simulink library "ammclib_bam_S32K11x"  (R2016a)
settings: Solver=VariableStepAuto  SolverMode=SingleTasking  StartTime=0.0  StopTime=10.0  RelTol=1e-3
undefined symbols (not defined in the file or in its folder): f16A1, f16A2, f16ADCMaxError, f16B0, f16B1, f16B2, f16C1, f16CC1, f16CC1sc, f16CC1sc_D, f16CC1sc_Q, f16CC2, f16CC2sc, f16CC2sc_D, f16CC2sc_Q, f16DerivGain, f16EGain, f16FiltCoef, f16HystOff, f16HystOn, f16IGain, f16IntegGain, f16IntegGainFW, f16IntegGainQ, f16Kd, f16Kq, f16Limit, f16LowerLimit, f16LowerLimit_D, f16LowerLimit_Q, f16LowerLimitFW, f16LowerLimitQ, f16ModIndex, f16OutValOff, f16OutValOn, f16PropGain, f16PropGainFW, f16PropGainQ, f16RampDown, f16RampUp, f16UGain, f16UpperLimit, f16UpperLimit_D, f16UpperLimit_Q, f16UpperLimitFW, f16UpperLimitQ, f16WIGain, f32A1, f32A2, f32ADCMaxError, f32B0, f32B1, f32B2, f32C1, f32CC1, f32CC1sc, f32CC1sc_D, f32CC1sc_Q, f32CC2, f32CC2sc ... (+62)
(part 15 of 16)

== system ammclib_bam_S32K11x/MLIB/F16/MLIB_VSub_F16 ==
  f16In1 : Inport  OutDataTypeStr=Bus: SWLIBS_2Syst_F16  BusOutputAsStruct=on
  f16In2 : Inport  Port=2  OutDataTypeStr=Bus: SWLIBS_2Syst_F16  BusOutputAsStruct=on
  MLIB_VSub_SF : S-Function  FunctionName=MLIB_VSub_SF_F16  SFunctionDeploymentMode=off  EnableBusSupport=off
  copyright : Subsystem
      mask Display: text(10,90,'FILE:');text(10,75,'DESRIPTION:');text(10,60,'COPYRIGHT:');text(10,45,'VERSION:');text(10,30,'DATE:')
  copyright2 : Subsystem
      mask Display: text(10,90,'MLIB_VSub_BAM_F16.mdl');text(10,75,'Vector substraction.');text(10,60,'NXP 2020');text(10,45,'1.0');text(10,30,'01-Jun-2020');
  f16Out : Outport
  wires:
  MLIB_VSub_SF/1 -> f16Out/1
  f16In2/1 -> MLIB_VSub_SF/2
  f16In1/1 -> MLIB_VSub_SF/1

== system ammclib_bam_S32K11x/MLIB/F32/MLIB_AbsSat_F32 ==
  f32In : Inport  OutDataTypeStr=int32
  MLIB_AbsSat_SF : S-Function  FunctionName=MLIB_AbsSat_SF_F32  SFunctionDeploymentMode=off  EnableBusSupport=off
  copyright : Subsystem
      mask Display: text(10,90,'FILE:');text(10,75,'DESRIPTION:');text(10,60,'COPYRIGHT:');text(10,45,'VERSION:');text(10,30,'DATE:')
  copyright2 : Subsystem
      mask Display: text(10,90,'MLIB_AbsSat_BAM_F32.mdl');text(10,75,'Saturated absolute value.');text(10,60,'NXP 2020');text(10,45,'1.0');text(10,30,'18-Mar-2020');
  f32Out : Outport
  wires:
  MLIB_AbsSat_SF/1 -> f32Out/1
  f32In/1 -> MLIB_AbsSat_SF/1

== system ammclib_bam_S32K11x/MLIB/F32/MLIB_Abs_F32 ==
  f32In : Inport  OutDataTypeStr=int32
  MLIB_Abs_SF : S-Function  FunctionName=MLIB_Abs_SF_F32  SFunctionDeploymentMode=off  EnableBusSupport=off
  copyright : Subsystem
      mask Display: text(10,90,'FILE:');text(10,75,'DESRIPTION:');text(10,60,'COPYRIGHT:');text(10,45,'VERSION:');text(10,30,'DATE:')
  copyright2 : Subsystem
      mask Display: text(10,90,'MLIB_Abs_BAM_F32.mdl');text(10,75,'Unsaturated absolute value.');text(10,60,'NXP 2020');text(10,45,'1.0');text(10,30,'18-Mar-2020');
  f32Out : Outport
  wires:
  MLIB_Abs_SF/1 -> f32Out/1
  f32In/1 -> MLIB_Abs_SF/1

== system ammclib_bam_S32K11x/MLIB/F32/MLIB_AddSat_F32 ==
  f32In1 : Inport  OutDataTypeStr=int32
  f32In2 : Inport  Port=2  OutDataTypeStr=int32
  MLIB_AddSat_SF : S-Function  FunctionName=MLIB_AddSat_SF_F32  SFunctionDeploymentMode=off  EnableBusSupport=off
  copyright : Subsystem
      mask Display: text(10,90,'FILE:');text(10,75,'DESRIPTION:');text(10,60,'COPYRIGHT:');text(10,45,'VERSION:');text(10,30,'DATE:')
  copyright2 : Subsystem
      mask Display: text(10,90,'MLIB_AddSat_BAM_F32.mdl');text(10,75,'Saturated addition.');text(10,60,'NXP 2020');text(10,45,'1.0');text(10,30,'18-Mar-2020');
  f32Out : Outport
  wires:
  MLIB_AddSat_SF/1 -> f32Out/1
  f32In2/1 -> MLIB_AddSat_SF/2
  f32In1/1 -> MLIB_AddSat_SF/1

== system ammclib_bam_S32K11x/MLIB/F32/MLIB_Add_F32 ==
  f32In1 : Inport  OutDataTypeStr=int32
  f32In2 : Inport  Port=2  OutDataTypeStr=int32
  MLIB_Add_SF : S-Function  FunctionName=MLIB_Add_SF_F32  SFunctionDeploymentMode=off  EnableBusSupport=off
  copyright : Subsystem
      mask Display: text(10,90,'FILE:');text(10,75,'DESRIPTION:');text(10,60,'COPYRIGHT:');text(10,45,'VERSION:');text(10,30,'DATE:')
  copyright2 : Subsystem
      mask Display: text(10,90,'MLIB_Add_BAM_F32.mdl');text(10,75,'Unsaturated addition.');text(10,60,'NXP 2020');text(10,45,'1.0');text(10,30,'18-Mar-2020');
  f32Out : Outport
  wires:
  MLIB_Add_SF/1 -> f32Out/1
  f32In2/1 -> MLIB_Add_SF/2
  f32In1/1 -> MLIB_Add_SF/1

== system ammclib_bam_S32K11x/MLIB/F32/MLIB_ConvertPU_F32F16 ==
  f16In : Inport  OutDataTypeStr=int16
  MLIB_ConvertPU_SF : S-Function  FunctionName=MLIB_ConvertPU_SF_F32F16  SFunctionDeploymentMode=off  EnableBusSupport=off
  copyright : Subsystem
      mask Display: text(10,90,'FILE:');text(10,75,'DESRIPTION:');text(10,60,'COPYRIGHT:');text(10,45,'VERSION:');text(10,30,'DATE:')
  copyright2 : Subsystem
      mask Display: text(10,90,'MLIB_ConvertPU_BAM_F32F16.mdl');text(10,75,'Converts the input value to a different representation.');text(10,60,'NXP 2020');text(10,45,'1.0');text(10,30,'18-Mar-2020');
  f32Out : Outport
  wires:
  MLIB_ConvertPU_SF/1 -> f32Out/1
  f16In/1 -> MLIB_ConvertPU_SF/1

== system ammclib_bam_S32K11x/MLIB/F32/MLIB_Convert_F32F16 ==
  f16In1 : Inport  OutDataTypeStr=int16
  f16In2 : Inport  Port=2  OutDataTypeStr=int16
  MLIB_Convert_SF : S-Function  FunctionName=MLIB_Convert_SF_F32F16  SFunctionDeploymentMode=off  EnableBusSupport=off
  copyright : Subsystem
      mask Display: text(10,90,'FILE:');text(10,75,'DESRIPTION:');text(10,60,'COPYRIGHT:');text(10,45,'VERSION:');text(10,30,'DATE:')
  copyright2 : Subsystem
      mask Display: text(10,90,'MLIB_Convert_BAM_F32F16.mdl');text(10,75,'Converts the input value with scale to a different representation.');text(10,60,'NXP 2020');text(10,45,'1.0');text(10,30,'18-Mar-2020');
  f32Out : Outport
  wires:
  MLIB_Convert_SF/1 -> f32Out/1
  f16In2/1 -> MLIB_Convert_SF/2
  f16In1/1 -> MLIB_Convert_SF/1

== system ammclib_bam_S32K11x/MLIB/F32/MLIB_DivSat_F32 ==
  f32In1 : Inport  OutDataTypeStr=int32
  f32In2 : Inport  Port=2  OutDataTypeStr=int32
  MLIB_DivSat_SF : S-Function  FunctionName=MLIB_DivSat_SF_F32  SFunctionDeploymentMode=off  EnableBusSupport=off
  copyright : Subsystem
      mask Display: text(10,90,'FILE:');text(10,75,'DESRIPTION:');text(10,60,'COPYRIGHT:');text(10,45,'VERSION:');text(10,30,'DATE:')
  copyright2 : Subsystem
      mask Display: text(10,90,'MLIB_DivSat_BAM_F32.mdl');text(10,75,'Saturated division.');text(10,60,'NXP 2020');text(10,45,'1.0');text(10,30,'18-Mar-2020');
  f32Out : Outport
  wires:
  MLIB_DivSat_SF/1 -> f32Out/1
  f32In2/1 -> MLIB_DivSat_SF/2
  f32In1/1 -> MLIB_DivSat_SF/1

== system ammclib_bam_S32K11x/MLIB/F32/MLIB_Div_F32 ==
  f32In1 : Inport  OutDataTypeStr=int32
  f32In2 : Inport  Port=2  OutDataTypeStr=int32
  MLIB_Div_SF : S-Function  FunctionName=MLIB_Div_SF_F32  SFunctionDeploymentMode=off  EnableBusSupport=off
  copyright : Subsystem
      mask Display: text(10,90,'FILE:');text(10,75,'DESRIPTION:');text(10,60,'COPYRIGHT:');text(10,45,'VERSION:');text(10,30,'DATE:')
  copyright2 : Subsystem
      mask Display: text(10,90,'MLIB_Div_BAM_F32.mdl');text(10,75,'Division of two input values.');text(10,60,'NXP 2020');text(10,45,'1.0');text(10,30,'18-Mar-2020');
  f32Out : Outport
  wires:
  MLIB_Div_SF/1 -> f32Out/1
  f32In2/1 -> MLIB_Div_SF/2
  f32In1/1 -> MLIB_Div_SF/1

== system ammclib_bam_S32K11x/MLIB/F32/MLIB_MacSat_F32 ==
  f32In1 : Inport  OutDataTypeStr=int32
  f32In2 : Inport  Port=2  OutDataTypeStr=int32
  f32In3 : Inport  Port=3  OutDataTypeStr=int32
  MLIB_MacSat_SF : S-Function  FunctionName=MLIB_MacSat_SF_F32  SFunctionDeploymentMode=off  EnableBusSupport=off
  copyright : Subsystem
      mask Display: text(10,90,'FILE:');text(10,75,'DESRIPTION:');text(10,60,'COPYRIGHT:');text(10,45,'VERSION:');text(10,30,'DATE:')
  copyright2 : Subsystem
      mask Display: text(10,90,'MLIB_MacSat_BAM_F32.mdl');text(10,75,'Saturated multiply-accumulate.');text(10,60,'NXP 2020');text(10,45,'1.0');text(10,30,'18-Mar-2020');
  f32Out : Outport
  wires:
  MLIB_MacSat_SF/1 -> f32Out/1
  f32In3/1 -> MLIB_MacSat_SF/3
  f32In2/1 -> MLIB_MacSat_SF/2
  f32In1/1 -> MLIB_MacSat_SF/1

== system ammclib_bam_S32K11x/MLIB/F32/MLIB_Mac_F32 ==
  f32In1 : Inport  OutDataTypeStr=int32
  f32In2 : Inport  Port=2  OutDataTypeStr=int32
  f32In3 : Inport  Port=3  OutDataTypeStr=int32
  MLIB_Mac_SF : S-Function  FunctionName=MLIB_Mac_SF_F32  SFunctionDeploymentMode=off  EnableBusSupport=off
  copyright : Subsystem
      mask Display: text(10,90,'FILE:');text(10,75,'DESRIPTION:');text(10,60,'COPYRIGHT:');text(10,45,'VERSION:');text(10,30,'DATE:')
  copyright2 : Subsystem
      mask Display: text(10,90,'MLIB_Mac_BAM_F32.mdl');text(10,75,'Multiply-accumulte.');text(10,60,'NXP 2020');text(10,45,'1.0');text(10,30,'18-Mar-2020');
  f32Out : Outport
  wires:
  MLIB_Mac_SF/1 -> f32Out/1
  f32In3/1 -> MLIB_Mac_SF/3
  f32In2/1 -> MLIB_Mac_SF/2
  f32In1/1 -> MLIB_Mac_SF/1

== system ammclib_bam_S32K11x/MLIB/F32/MLIB_Mnac_F32 ==
  f32In1 : Inport  OutDataTypeStr=int32
  f32In2 : Inport  Port=2  OutDataTypeStr=int32
  f32In3 : Inport  Port=3  OutDataTypeStr=int32
  MLIB_Mnac_SF : S-Function  FunctionName=MLIB_Mnac_SF_F32  SFunctionDeploymentMode=off  EnableBusSupport=off
  copyright : Subsystem
      mask Display: text(10,90,'FILE:');text(10,75,'DESRIPTION:');text(10,60,'COPYRIGHT:');text(10,45,'VERSION:');text(10,30,'DATE:')
  copyright2 : Subsystem
      mask Display: text(10,90,'MLIB_Mnac_BAM_F32.mdl');text(10,75,'Unsaturated multiply-negative-accumulate.');text(10,60,'NXP 2020');text(10,45,'1.0');text(10,30,'18-Mar-2020');
  f32Out : Outport
  wires:
  MLIB_Mnac_SF/1 -> f32Out/1
  f32In3/1 -> MLIB_Mnac_SF/3
  f32In2/1 -> MLIB_Mnac_SF/2
  f32In1/1 -> MLIB_Mnac_SF/1

== system ammclib_bam_S32K11x/MLIB/F32/MLIB_Msu_F32 ==
  f32In1 : Inport  OutDataTypeStr=int32
  f32In2 : Inport  Port=2  OutDataTypeStr=int32
  f32In3 : Inport  Port=3  OutDataTypeStr=int32
  MLIB_Msu_SF : S-Function  FunctionName=MLIB_Msu_SF_F32  SFunctionDeploymentMode=off  EnableBusSupport=off
  copyright : Subsystem
      mask Display: text(10,90,'FILE:');text(10,75,'DESRIPTION:');text(10,60,'COPYRIGHT:');text(10,45,'VERSION:');text(10,30,'DATE:')
  copyright2 : Subsystem
      mask Display: text(10,90,'MLIB_Msu_BAM_F32.mdl');text(10,75,'Unsaturated multiply-subtract-from.');text(10,60,'NXP 2020');text(10,45,'1.0');text(10,30,'18-Mar-2020');
  f32Out : Outport
  wires:
  MLIB_Msu_SF/1 -> f32Out/1
  f32In3/1 -> MLIB_Msu_SF/3
  f32In2/1 -> MLIB_Msu_SF/2
  f32In1/1 -> MLIB_Msu_SF/1

== system ammclib_bam_S32K11x/MLIB/F32/MLIB_MulSat_F32 ==
  f32In1 : Inport  OutDataTypeStr=int32
  f32In2 : Inport  Port=2  OutDataTypeStr=int32
  MLIB_MulSat_SF : S-Function  FunctionName=MLIB_MulSat_SF_F32  SFunctionDeploymentMode=off  EnableBusSupport=off
  copyright : Subsystem
      mask Display: text(10,90,'FILE:');text(10,75,'DESRIPTION:');text(10,60,'COPYRIGHT:');text(10,45,'VERSION:');text(10,30,'DATE:')
  copyright2 : Subsystem
      mask Display: text(10,90,'MLIB_MulSat_BAM_F32.mdl');text(10,75,'Saturated multiplication.');text(10,60,'NXP 2020');text(10,45,'1.0');text(10,30,'18-Mar-2020');
  f32Out : Outport
  wires:
  MLIB_MulSat_SF/1 -> f32Out/1
  f32In2/1 -> MLIB_MulSat_SF/2
  f32In1/1 -> MLIB_MulSat_SF/1

== system ammclib_bam_S32K11x/MLIB/F32/MLIB_Mul_F32 ==
  f32In1 : Inport  OutDataTypeStr=int32
  f32In2 : Inport  Port=2  OutDataTypeStr=int32
  MLIB_Mul_SF : S-Function  FunctionName=MLIB_Mul_SF_F32  SFunctionDeploymentMode=off  EnableBusSupport=off
  copyright : Subsystem
      mask Display: text(10,90,'FILE:');text(10,75,'DESRIPTION:');text(10,60,'COPYRIGHT:');text(10,45,'VERSION:');text(10,30,'DATE:')
  copyright2 : Subsystem
      mask Display: text(10,90,'MLIB_Mul_BAM_F32.mdl');text(10,75,'Unsaturated multiplication.');text(10,60,'NXP 2020');text(10,45,'1.0');text(10,30,'18-Mar-2020');
  f32Out : Outport
  wires:
  MLIB_Mul_SF/1 -> f32Out/1
  f32In2/1 -> MLIB_Mul_SF/2
  f32In1/1 -> MLIB_Mul_SF/1

== system ammclib_bam_S32K11x/MLIB/F32/MLIB_NegSat_F32 ==
  f32In : Inport  OutDataTypeStr=int32
  MLIB_NegSat_SF : S-Function  FunctionName=MLIB_NegSat_SF_F32  SFunctionDeploymentMode=off  EnableBusSupport=off
  copyright : Subsystem
      mask Display: text(10,90,'FILE:');text(10,75,'DESRIPTION:');text(10,60,'COPYRIGHT:');text(10,45,'VERSION:');text(10,30,'DATE:')
  copyright2 : Subsystem
      mask Display: text(10,90,'MLIB_NegSat_BAM_F32.mdl');text(10,75,'Saturated negation.');text(10,60,'NXP 2020');text(10,45,'1.0');text(10,30,'18-Mar-2020');
  f32Out : Outport
  wires:
  MLIB_NegSat_SF/1 -> f32Out/1
  f32In/1 -> MLIB_NegSat_SF/1

== system ammclib_bam_S32K11x/MLIB/F32/MLIB_Neg_F32 ==
  f32In : Inport  OutDataTypeStr=int32
  MLIB_Neg_SF : S-Function  FunctionName=MLIB_Neg_SF_F32  SFunctionDeploymentMode=off  EnableBusSupport=off
  copyright : Subsystem
      mask Display: text(10,90,'FILE:');text(10,75,'DESRIPTION:');text(10,60,'COPYRIGHT:');text(10,45,'VERSION:');text(10,30,'DATE:')
  copyright2 : Subsystem
      mask Display: text(10,90,'MLIB_Neg_BAM_F32.mdl');text(10,75,'Unsaturated negation.');text(10,60,'NXP 2020');text(10,45,'1.0');text(10,30,'18-Mar-2020');
  f32Out : Outport
  wires:
  MLIB_Neg_SF/1 -> f32Out/1
  f32In/1 -> MLIB_Neg_SF/1

== system ammclib_bam_S32K11x/MLIB/F32/MLIB_Norm_F32 ==
  f32In : Inport  OutDataTypeStr=int32
  MLIB_Norm_SF : S-Function  FunctionName=MLIB_Norm_SF_F32  SFunctionDeploymentMode=off  EnableBusSupport=off
  copyright : Subsystem
      mask Display: text(10,90,'FILE:');text(10,75,'DESRIPTION:');text(10,60,'COPYRIGHT:');text(10,45,'VERSION:');text(10,30,'DATE:')
  copyright2 : Subsystem
      mask Display: text(10,90,'MLIB_Norm_BAM_F32.mdl');text(10,75,'Normalization of the input value.');text(10,60,'NXP 2020');text(10,45,'1.0');text(10,30,'18-Mar-2020');
  u16Out : Outport
  wires:
  MLIB_Norm_SF/1 -> u16Out/1
  f32In/1 -> MLIB_Norm_SF/1

== system ammclib_bam_S32K11x/MLIB/F32/MLIB_Round_F32 ==
  f32In1 : Inport  OutDataTypeStr=int32
  u16In2 : Inport  Port=2  OutDataTypeStr=uint16
  MLIB_Round_SF : S-Function  FunctionName=MLIB_Round_SF_F32  SFunctionDeploymentMode=off  EnableBusSupport=off
  copyright : Subsystem
      mask Display: text(10,90,'FILE:');text(10,75,'DESRIPTION:');text(10,60,'COPYRIGHT:');text(10,45,'VERSION:');text(10,30,'DATE:')
  copyright2 : Subsystem
      mask Display: text(10,90,'MLIB_Round_BAM_F32.mdl');text(10,75,'Round the first input value.');text(10,60,'NXP 2020');text(10,45,'1.0');text(10,30,'18-Mar-2020');
  f32Out : Outport
  wires:
  MLIB_Round_SF/1 -> f32Out/1
  u16In2/1 -> MLIB_Round_SF/2
  f32In1/1 -> MLIB_Round_SF/1

== system ammclib_bam_S32K11x/MLIB/F32/MLIB_ShBiSat_F32 ==
  f32In1 : Inport  OutDataTypeStr=int32
  s16In2 : Inport  Port=2  OutDataTypeStr=int16
  MLIB_ShBiSat_SF : S-Function  FunctionName=MLIB_ShBiSat_SF_F32  SFunctionDeploymentMode=off  EnableBusSupport=off
  copyright : Subsystem
      mask Display: text(10,90,'FILE:');text(10,75,'DESRIPTION:');text(10,60,'COPYRIGHT:');text(10,45,'VERSION:');text(10,30,'DATE:')
  copyright2 : Subsystem
      mask Display: text(10,90,'MLIB_ShBiSat_BAM_F32.mdl');text(10,75,'Saturated bidirectional shift.');text(10,60,'NXP 2020');text(10,45,'1.0');text(10,30,'18-Mar-2020');
  f32Out : Outport
  wires:
  MLIB_ShBiSat_SF/1 -> f32Out/1
  s16In2/1 -> MLIB_ShBiSat_SF/2
  f32In1/1 -> MLIB_ShBiSat_SF/1

== system ammclib_bam_S32K11x/MLIB/F32/MLIB_ShBi_F32 ==
  f32In1 : Inport  OutDataTypeStr=int32
  s16In2 : Inport  Port=2  OutDataTypeStr=int16
  MLIB_ShBi_SF : S-Function  FunctionName=MLIB_ShBi_SF_F32  SFunctionDeploymentMode=off  EnableBusSupport=off
  copyright : Subsystem
      mask Display: text(10,90,'FILE:');text(10,75,'DESRIPTION:');text(10,60,'COPYRIGHT:');text(10,45,'VERSION:');text(10,30,'DATE:')
  copyright2 : Subsystem
      mask Display: text(10,90,'MLIB_ShBi_BAM_F32.mdl');text(10,75,'Unsaturated bidirectional shift.');text(10,60,'NXP 2020');text(10,45,'1.0');text(10,30,'18-Mar-2020');
  f32Out : Outport
  wires:
  MLIB_ShBi_SF/1 -> f32Out/1
  s16In2/1 -> MLIB_ShBi_SF/2
  f32In1/1 -> MLIB_ShBi_SF/1

== system ammclib_bam_S32K11x/MLIB/F32/MLIB_ShLSat_F32 ==
  f32In1 : Inport  OutDataTypeStr=int32
  u16In2 : Inport  Port=2  OutDataTypeStr=uint16
  MLIB_ShLSat_SF : S-Function  FunctionName=MLIB_ShLSat_SF_F32  SFunctionDeploymentMode=off  EnableBusSupport=off
  copyright : Subsystem
      mask Display: text(10,90,'FILE:');text(10,75,'DESRIPTION:');text(10,60,'COPYRIGHT:');text(10,45,'VERSION:');text(10,30,'DATE:')
  copyright2 : Subsystem
      mask Display: text(10,90,'MLIB_ShLSat_BAM_F32.mdl');text(10,75,'Saturated shift left.');text(10,60,'NXP 2020');text(10,45,'1.0');text(10,30,'18-Mar-2020');
  f32Out : Outport
  wires:
  MLIB_ShLSat_SF/1 -> f32Out/1
  u16In2/1 -> MLIB_ShLSat_SF/2
  f32In1/1 -> MLIB_ShLSat_SF/1

== system ammclib_bam_S32K11x/MLIB/F32/MLIB_ShL_F32 ==
  f32In1 : Inport  OutDataTypeStr=int32
  u16In2 : Inport  Port=2  OutDataTypeStr=uint16
  MLIB_ShL_SF : S-Function  FunctionName=MLIB_ShL_SF_F32  SFunctionDeploymentMode=off  EnableBusSupport=off
  copyright : Subsystem
      mask Display: text(10,90,'FILE:');text(10,75,'DESRIPTION:');text(10,60,'COPYRIGHT:');text(10,45,'VERSION:');text(10,30,'DATE:')
  copyright2 : Subsystem
      mask Display: text(10,90,'MLIB_ShL_BAM_F32.mdl');text(10,75,'Unsaturated shift left.');text(10,60,'NXP 2020');text(10,45,'1.0');text(10,30,'18-Mar-2020');
  f32Out : Outport
  wires:
  MLIB_ShL_SF/1 -> f32Out/1
  u16In2/1 -> MLIB_ShL_SF/2
  f32In1/1 -> MLIB_ShL_SF/1

== system ammclib_bam_S32K11x/MLIB/F32/MLIB_ShR_F32 ==
  f32In1 : Inport  OutDataTypeStr=int32
  u16In2 : Inport  Port=2  OutDataTypeStr=uint16
  MLIB_ShR_SF : S-Function  FunctionName=MLIB_ShR_SF_F32  SFunctionDeploymentMode=off  EnableBusSupport=off
  copyright : Subsystem
      mask Display: text(10,90,'FILE:');text(10,75,'DESRIPTION:');text(10,60,'COPYRIGHT:');text(10,45,'VERSION:');text(10,30,'DATE:')
  copyright2 : Subsystem
      mask Display: text(10,90,'MLIB_ShR_BAM_F32.mdl');text(10,75,'Unsaturated shift right.');text(10,60,'NXP 2020');text(10,45,'1.0');text(10,30,'18-Mar-2020');
  f32Out : Outport
  wires:
  MLIB_ShR_SF/1 -> f32Out/1
  u16In2/1 -> MLIB_ShR_SF/2
  f32In1/1 -> MLIB_ShR_SF/1

== system ammclib_bam_S32K11x/MLIB/F32/MLIB_SubSat_F32 ==
  f32In1 : Inport  OutDataTypeStr=int32
  f32In2 : Inport  Port=2  OutDataTypeStr=int32
  MLIB_SubSat_SF : S-Function  FunctionName=MLIB_SubSat_SF_F32  SFunctionDeploymentMode=off  EnableBusSupport=off
  copyright : Subsystem
      mask Display: text(10,90,'FILE:');text(10,75,'DESRIPTION:');text(10,60,'COPYRIGHT:');text(10,45,'VERSION:');text(10,30,'DATE:')
  copyright2 : Subsystem
      mask Display: text(10,90,'MLIB_SubSat_BAM_F32.mdl');text(10,75,'Saturated subtraction.');text(10,60,'NXP 2020');text(10,45,'1.0');text(10,30,'18-Mar-2020');
  f32Out : Outport
  wires:
  MLIB_SubSat_SF/1 -> f32Out/1
  f32In2/1 -> MLIB_SubSat_SF/2
  f32In1/1 -> MLIB_SubSat_SF/1

== system ammclib_bam_S32K11x/MLIB/F32/MLIB_Sub_F32 ==
  f32In1 : Inport  OutDataTypeStr=int32
  f32In2 : Inport  Port=2  OutDataTypeStr=int32
  MLIB_Sub_SF : S-Function  FunctionName=MLIB_Sub_SF_F32  SFunctionDeploymentMode=off  EnableBusSupport=off
  copyright : Subsystem
      mask Display: text(10,90,'FILE:');text(10,75,'DESRIPTION:');text(10,60,'COPYRIGHT:');text(10,45,'VERSION:');text(10,30,'DATE:')
  copyright2 : Subsystem
      mask Display: text(10,90,'MLIB_Sub_BAM_F32.mdl');text(10,75,'Unsaturated subtraction.');text(10,60,'NXP 2020');text(10,45,'1.0');text(10,30,'18-Mar-2020');
  f32Out : Outport
  wires:
  MLIB_Sub_SF/1 -> f32Out/1
  f32In2/1 -> MLIB_Sub_SF/2
  f32In1/1 -> MLIB_Sub_SF/1

== system ammclib_bam_S32K11x/MLIB/F32/MLIB_VAdd_F32 ==
  f32In1 : Inport  OutDataTypeStr=Bus: SWLIBS_2Syst_F32  BusOutputAsStruct=on
  f32In2 : Inport  Port=2  OutDataTypeStr=Bus: SWLIBS_2Syst_F32  BusOutputAsStruct=on
  MLIB_VAdd_SF : S-Function  FunctionName=MLIB_VAdd_SF_F32  SFunctionDeploymentMode=off  EnableBusSupport=off
  copyright : Subsystem
      mask Display: text(10,90,'FILE:');text(10,75,'DESRIPTION:');text(10,60,'COPYRIGHT:');text(10,45,'VERSION:');text(10,30,'DATE:')
  copyright2 : Subsystem
      mask Display: text(10,90,'MLIB_VAdd_BAM_F32.mdl');text(10,75,'Vector addition.');text(10,60,'NXP 2020');text(10,45,'1.0');text(10,30,'28-May-2020');
  f32Out : Outport
  wires:
  MLIB_VAdd_SF/1 -> f32Out/1
  f32In2/1 -> MLIB_VAdd_SF/2
  f32In1/1 -> MLIB_VAdd_SF/1

== system ammclib_bam_S32K11x/MLIB/F32/MLIB_VMac_F32 ==
  f32In1 : Inport  OutDataTypeStr=int32
  f32In2 : Inport  Port=2  OutDataTypeStr=int32
  f32In3 : Inport  Port=3  OutDataTypeStr=int32
  f32In4 : Inport  Port=4  OutDataTypeStr=int32
  MLIB_VMac_SF : S-Function  FunctionName=MLIB_VMac_SF_F32  SFunctionDeploymentMode=off  EnableBusSupport=off
  copyright : Subsystem
      mask Display: text(10,90,'FILE:');text(10,75,'DESRIPTION:');text(10,60,'COPYRIGHT:');text(10,45,'VERSION:');text(10,30,'DATE:')
  copyright2 : Subsystem
      mask Display: text(10,90,'MLIB_VMac_BAM_F32.mdl');text(10,75,'Dot product of 2-element vectors with saturated multiplication and modulo accumulation.');text(10,60,'NXP 2020');text(10,45,'1.0');text(10,30,'18-Mar-2020');
  f32Out : Outport
  wires:
  MLIB_VMac_SF/1 -> f32Out/1
  f32In4/1 -> MLIB_VMac_SF/4
  f32In3/1 -> MLIB_VMac_SF/3
  f32In2/1 -> MLIB_VMac_SF/2
  f32In1/1 -> MLIB_VMac_SF/1

== system ammclib_bam_S32K11x/MLIB/F32/MLIB_VScale_F32 ==
  f32InVec : Inport  OutDataTypeStr=Bus: SWLIBS_2Syst_F32  BusOutputAsStruct=on
  f32InScale : Inport  Port=2  OutDataTypeStr=int32
  MLIB_VScale_SF : S-Function  FunctionName=MLIB_VScale_SF_F32  SFunctionDeploymentMode=off  EnableBusSupport=off
  copyright : Subsystem
      mask Display: text(10,90,'FILE:');text(10,75,'DESRIPTION:');text(10,60,'COPYRIGHT:');text(10,45,'VERSION:');text(10,30,'DATE:')
  copyright2 : Subsystem
      mask Display: text(10,90,'MLIB_VScale_BAM_F32.mdl');text(10,75,'Multiplication of a vector and scalar.');text(10,60,'NXP 2020');text(10,45,'1.0');text(10,30,'03-Jun-2020');
  f32OutVec : Outport
  wires:
  MLIB_VScale_SF/1 -> f32OutVec/1
  f32InScale/1 -> MLIB_VScale_SF/2
  f32InVec/1 -> MLIB_VScale_SF/1

== system ammclib_bam_S32K11x/MLIB/F32/MLIB_VSub_F32 ==
  f32In1 : Inport  OutDataTypeStr=Bus: SWLIBS_2Syst_F32  BusOutputAsStruct=on
  f32In2 : Inport  Port=2  OutDataTypeStr=Bus: SWLIBS_2Syst_F32  BusOutputAsStruct=on
  MLIB_VSub_SF : S-Function  FunctionName=MLIB_VSub_SF_F32  SFunctionDeploymentMode=off  EnableBusSupport=off
  copyright : Subsystem
      mask Display: text(10,90,'FILE:');text(10,75,'DESRIPTION:');text(10,60,'COPYRIGHT:');text(10,45,'VERSION:');text(10,30,'DATE:')
  copyright2 : Subsystem
      mask Display: text(10,90,'MLIB_VSub_BAM_F32.mdl');text(10,75,'Vector substraction.');text(10,60,'NXP 2020');text(10,45,'1.0');text(10,30,'01-Jun-2020');
  f32Out : Outport
  wires:
  MLIB_VSub_SF/1 -> f32Out/1
  f32In2/1 -> MLIB_VSub_SF/2
  f32In1/1 -> MLIB_VSub_SF/1

== system ammclib_bam_S32K11x/MLIB/F32F16F16/MLIB_MacSat_F32F16F16 ==
  f32In1 : Inport  OutDataTypeStr=int32
  f16In2 : Inport  Port=2  OutDataTypeStr=int16
  f16In3 : Inport  Port=3  OutDataTypeStr=int16
  MLIB_MacSat_SF : S-Function  FunctionName=MLIB_MacSat_SF_F32F16F16  SFunctionDeploymentMode=off  EnableBusSupport=off
  copyright : Subsystem
      mask Display: text(10,90,'FILE:');text(10,75,'DESRIPTION:');text(10,60,'COPYRIGHT:');text(10,45,'VERSION:');text(10,30,'DATE:')
  copyright2 : Subsystem
      mask Display: text(10,90,'MLIB_MacSat_BAM_F32F16F16.mdl');text(10,75,'Saturated multiply-accumulate.');text(10,60,'NXP 2020');text(10,45,'1.0');text(10,30,'18-Mar-2020');
  f32Out : Outport
  wires:
  MLIB_MacSat_SF/1 -> f32Out/1
  f16In3/1 -> MLIB_MacSat_SF/3
  f16In2/1 -> MLIB_MacSat_SF/2
  f32In1/1 -> MLIB_MacSat_SF/1

== system ammclib_bam_S32K11x/MLIB/F32F16F16/MLIB_Mac_F32F16F16 ==
  f32In1 : Inport  OutDataTypeStr=int32
  f16In2 : Inport  Port=2  OutDataTypeStr=int16
  f16In3 : Inport  Port=3  OutDataTypeStr=int16
  MLIB_Mac_SF : S-Function  FunctionName=MLIB_Mac_SF_F32F16F16  SFunctionDeploymentMode=off  EnableBusSupport=off
  copyright : Subsystem
      mask Display: text(10,90,'FILE:');text(10,75,'DESRIPTION:');text(10,60,'COPYRIGHT:');text(10,45,'VERSION:');text(10,30,'DATE:')
  copyright2 : Subsystem
      mask Display: text(10,90,'MLIB_Mac_BAM_F32F16F16.mdl');text(10,75,'Multiply-accumulte.');text(10,60,'NXP 2020');text(10,45,'1.0');text(10,30,'18-Mar-2020');
  f32Out : Outport
  wires:
  MLIB_Mac_SF/1 -> f32Out/1
  f16In3/1 -> MLIB_Mac_SF/3
  f16In2/1 -> MLIB_Mac_SF/2
  f32In1/1 -> MLIB_Mac_SF/1

== system ammclib_bam_S32K11x/MLIB/F32F16F16/MLIB_Mnac_F32F16F16 ==
  f32In1 : Inport  OutDataTypeStr=int32
  f16In2 : Inport  Port=2  OutDataTypeStr=int16
  f16In3 : Inport  Port=3  OutDataTypeStr=int16
  MLIB_Mnac_SF : S-Function  FunctionName=MLIB_Mnac_SF_F32F16F16  SFunctionDeploymentMode=off  EnableBusSupport=off
  copyright : Subsystem
      mask Display: text(10,90,'FILE:');text(10,75,'DESRIPTION:');text(10,60,'COPYRIGHT:');text(10,45,'VERSION:');text(10,30,'DATE:')
  copyright2 : Subsystem
      mask Display: text(10,90,'MLIB_Mnac_BAM_F32F16F16.mdl');text(10,75,'Unsaturated multiply-negative-accumulate.');text(10,60,'NXP 2020');text(10,45,'1.0');text(10,30,'18-Mar-2020');
  f32Out : Outport
  wires:
  MLIB_Mnac_SF/1 -> f32Out/1
  f16In3/1 -> MLIB_Mnac_SF/3
  f16In2/1 -> MLIB_Mnac_SF/2
  f32In1/1 -> MLIB_Mnac_SF/1

== system ammclib_bam_S32K11x/MLIB/F32F16F16/MLIB_Msu_F32F16F16 ==
  f32In1 : Inport  OutDataTypeStr=int32
  f16In2 : Inport  Port=2  OutDataTypeStr=int16
  f16In3 : Inport  Port=3  OutDataTypeStr=int16
  MLIB_Msu_SF : S-Function  FunctionName=MLIB_Msu_SF_F32F16F16  SFunctionDeploymentMode=off  EnableBusSupport=off
  copyright : Subsystem
      mask Display: text(10,90,'FILE:');text(10,75,'DESRIPTION:');text(10,60,'COPYRIGHT:');text(10,45,'VERSION:');text(10,30,'DATE:')
  copyright2 : Subsystem
      mask Display: text(10,90,'MLIB_Msu_BAM_F32F16F16.mdl');text(10,75,'Unsaturated multiply-subtract-from.');text(10,60,'NXP 2020');text(10,45,'1.0');text(10,30,'18-Mar-2020');
  f32Out : Outport
  wires:
  MLIB_Msu_SF/1 -> f32Out/1
  f16In3/1 -> MLIB_Msu_SF/3
  f16In2/1 -> MLIB_Msu_SF/2
  f32In1/1 -> MLIB_Msu_SF/1

== system ammclib_bam_S32K11x/MLIB/F32F16F16/MLIB_MulSat_F32F16F16 ==
  f16In1 : Inport  OutDataTypeStr=int16
  f16In2 : Inport  Port=2  OutDataTypeStr=int16
  MLIB_MulSat_SF : S-Function  FunctionName=MLIB_MulSat_SF_F32F16F16  SFunctionDeploymentMode=off  EnableBusSupport=off
  copyright : Subsystem
      mask Display: text(10,90,'FILE:');text(10,75,'DESRIPTION:');text(10,60,'COPYRIGHT:');text(10,45,'VERSION:');text(10,30,'DATE:')
  copyright2 : Subsystem
      mask Display: text(10,90,'MLIB_MulSat_BAM_F32F16F16.mdl');text(10,75,'Saturated multiplication.');text(10,60,'NXP 2020');text(10,45,'1.0');text(10,30,'18-Mar-2020');
  f32Out : Outport
  wires:
  MLIB_MulSat_SF/1 -> f32Out/1
  f16In2/1 -> MLIB_MulSat_SF/2
  f16In1/1 -> MLIB_MulSat_SF/1

== system ammclib_bam_S32K11x/MLIB/F32F16F16/MLIB_Mul_F32F16F16 ==
  f16In1 : Inport  OutDataTypeStr=int16
  f16In2 : Inport  Port=2  OutDataTypeStr=int16
  MLIB_Mul_SF : S-Function  FunctionName=MLIB_Mul_SF_F32F16F16  SFunctionDeploymentMode=off  EnableBusSupport=off
  copyright : Subsystem
      mask Display: text(10,90,'FILE:');text(10,75,'DESRIPTION:');text(10,60,'COPYRIGHT:');text(10,45,'VERSION:');text(10,30,'DATE:')
  copyright2 : Subsystem
      mask Display: text(10,90,'MLIB_Mul_BAM_F32F16F16.mdl');text(10,75,'Unsaturated multiplication.');text(10,60,'NXP 2020');text(10,45,'1.0');text(10,30,'18-Mar-2020');
  f32Out : Outport
  wires:
  MLIB_Mul_SF/1 -> f32Out/1
  f16In2/1 -> MLIB_Mul_SF/2
  f16In1/1 -> MLIB_Mul_SF/1

== system ammclib_bam_S32K11x/MLIB/F32F16F16/MLIB_VMac_F32F16F16 ==
  f16In1 : Inport  OutDataTypeStr=int16
  f16In2 : Inport  Port=2  OutDataTypeStr=int16
  f16In3 : Inport  Port=3  OutDataTypeStr=int16
  f16In4 : Inport  Port=4  OutDataTypeStr=int16
  MLIB_VMac_SF : S-Function  FunctionName=MLIB_VMac_SF_F32F16F16  SFunctionDeploymentMode=off  EnableBusSupport=off
  copyright : Subsystem
      mask Display: text(10,90,'FILE:');text(10,75,'DESRIPTION:');text(10,60,'COPYRIGHT:');text(10,45,'VERSION:');text(10,30,'DATE:')
  copyright2 : Subsystem
      mask Display: text(10,90,'MLIB_VMac_BAM_F32F16F16.mdl');text(10,75,'Dot product of 2-element vectors with saturated multiplication and modulo accumulation.');text(10,60,'NXP 2020');text(10,45,'1.0');text(10,30,'18-Mar-2020');
  f32Out : Outport
  wires:
  MLIB_VMac_SF/1 -> f32Out/1
  f16In4/1 -> MLIB_VMac_SF/4
  f16In3/1 -> MLIB_VMac_SF/3
  f16In2/1 -> MLIB_VMac_SF/2
  f16In1/1 -> MLIB_VMac_SF/1

== system ammclib_bam_S32K11x/AMCLIB/F16/AMCLIB_BemfObsrvDQ_F16/copyright ==

== system ammclib_bam_S32K11x/AMCLIB/F16/AMCLIB_BemfObsrvDQ_F16/copyright2 ==

== system ammclib_bam_S32K11x/AMCLIB/F16/AMCLIB_CurrentLoop_F16/copyright ==

== system ammclib_bam_S32K11x/AMCLIB/F16/AMCLIB_CurrentLoop_F16/copyright2 ==

== system ammclib_bam_S32K11x/AMCLIB/F16/AMCLIB_FWSpeedLoop_F16/copyright ==

== system ammclib_bam_S32K11x/AMCLIB/F16/AMCLIB_FWSpeedLoop_F16/copyright2 ==

== system ammclib_bam_S32K11x/AMCLIB/F16/AMCLIB_FW_F16/copyright ==

== system ammclib_bam_S32K11x/AMCLIB/F16/AMCLIB_FW_F16/copyright2 ==

== system ammclib_bam_S32K11x/AMCLIB/F16/AMCLIB_SpeedLoop_F16/copyright ==

== system ammclib_bam_S32K11x/AMCLIB/F16/AMCLIB_SpeedLoop_F16/copyright2 ==

== system ammclib_bam_S32K11x/AMCLIB/F16/AMCLIB_TrackObsrv_F16/copyright ==

== system ammclib_bam_S32K11x/AMCLIB/F16/AMCLIB_TrackObsrv_F16/copyright2 ==

== system ammclib_bam_S32K11x/AMCLIB/F16/AMCLIB_Windmilling_F16/copyright ==

== system ammclib_bam_S32K11x/AMCLIB/F16/AMCLIB_Windmilling_F16/copyright2 ==

== system ammclib_bam_S32K11x/AMCLIB/F32/AMCLIB_BemfObsrvDQ_F32/copyright ==

== system ammclib_bam_S32K11x/AMCLIB/F32/AMCLIB_BemfObsrvDQ_F32/copyright2 ==

== system ammclib_bam_S32K11x/AMCLIB/F32/AMCLIB_CurrentLoop_F32/copyright ==

== system ammclib_bam_S32K11x/AMCLIB/F32/AMCLIB_CurrentLoop_F32/copyright2 ==

== system ammclib_bam_S32K11x/AMCLIB/F32/AMCLIB_FWSpeedLoop_F32/copyright ==

== system ammclib_bam_S32K11x/AMCLIB/F32/AMCLIB_FWSpeedLoop_F32/copyright2 ==

== system ammclib_bam_S32K11x/AMCLIB/F32/AMCLIB_FW_F32/copyright ==

== system ammclib_bam_S32K11x/AMCLIB/F32/AMCLIB_FW_F32/copyright2 ==

== system ammclib_bam_S32K11x/AMCLIB/F32/AMCLIB_SpeedLoop_F32/copyright ==

== system ammclib_bam_S32K11x/AMCLIB/F32/AMCLIB_SpeedLoop_F32/copyright2 ==

== system ammclib_bam_S32K11x/AMCLIB/F32/AMCLIB_TrackObsrv_F32/copyright ==

== system ammclib_bam_S32K11x/AMCLIB/F32/AMCLIB_TrackObsrv_F32/copyright2 ==

== system ammclib_bam_S32K11x/AMCLIB/F32/AMCLIB_Windmilling_F32/copyright ==

== system ammclib_bam_S32K11x/AMCLIB/F32/AMCLIB_Windmilling_F32/copyright2 ==

== system ammclib_bam_S32K11x/GDFLIB/F16/GDFLIB_FilterFIR_F16/copyright ==

== system ammclib_bam_S32K11x/GDFLIB/F16/GDFLIB_FilterFIR_F16/copyright2 ==

== system ammclib_bam_S32K11x/GDFLIB/F16/GDFLIB_FilterIIR1_F16/copyright ==

== system ammclib_bam_S32K11x/GDFLIB/F16/GDFLIB_FilterIIR1_F16/copyright2 ==

== system ammclib_bam_S32K11x/GDFLIB/F16/GDFLIB_FilterIIR2_F16/copyright ==

== system ammclib_bam_S32K11x/GDFLIB/F16/GDFLIB_FilterIIR2_F16/copyright2 ==

== system ammclib_bam_S32K11x/GDFLIB/F16/GDFLIB_FilterMA_F16/copyright ==

== system ammclib_bam_S32K11x/GDFLIB/F16/GDFLIB_FilterMA_F16/copyright2 ==

== system ammclib_bam_S32K11x/GDFLIB/F32/GDFLIB_FilterFIR_F32/copyright ==

== system ammclib_bam_S32K11x/GDFLIB/F32/GDFLIB_FilterFIR_F32/copyright2 ==

== system ammclib_bam_S32K11x/GDFLIB/F32/GDFLIB_FilterIIR1_F32/copyright ==

== system ammclib_bam_S32K11x/GDFLIB/F32/GDFLIB_FilterIIR1_F32/copyright2 ==

== system ammclib_bam_S32K11x/GDFLIB/F32/GDFLIB_FilterIIR2_F32/copyright ==

== system ammclib_bam_S32K11x/GDFLIB/F32/GDFLIB_FilterIIR2_F32/copyright2 ==

== system ammclib_bam_S32K11x/GDFLIB/F32/GDFLIB_FilterMA_F32/copyright ==

== system ammclib_bam_S32K11x/GDFLIB/F32/GDFLIB_FilterMA_F32/copyright2 ==

== system ammclib_bam_S32K11x/GFLIB/F16/GFLIB_Acos_F16/copyright ==

== system ammclib_bam_S32K11x/GFLIB/F16/GFLIB_Acos_F16/copyright2 ==

== system ammclib_bam_S32K11x/GFLIB/F16/GFLIB_Asin_F16/copyright ==

== system ammclib_bam_S32K11x/GFLIB/F16/GFLIB_Asin_F16/copyright2 ==

== system ammclib_bam_S32K11x/GFLIB/F16/GFLIB_AtanYXShifted_F16/copyright ==

== system ammclib_bam_S32K11x/GFLIB/F16/GFLIB_AtanYXShifted_F16/copyright2 ==

== system ammclib_bam_S32K11x/GFLIB/F16/GFLIB_AtanYX_F16/copyright ==

== system ammclib_bam_S32K11x/GFLIB/F16/GFLIB_AtanYX_F16/copyright2 ==

== system ammclib_bam_S32K11x/GFLIB/F16/GFLIB_Atan_F16/copyright ==

== system ammclib_bam_S32K11x/GFLIB/F16/GFLIB_Atan_F16/copyright2 ==

== system ammclib_bam_S32K11x/GFLIB/F16/GFLIB_ControllerPIDpAW_F16/copyright ==

== system ammclib_bam_S32K11x/GFLIB/F16/GFLIB_ControllerPIDpAW_F16/copyright2 ==

== system ammclib_bam_S32K11x/GFLIB/F16/GFLIB_ControllerPIpAW_F16/copyright ==

== system ammclib_bam_S32K11x/GFLIB/F16/GFLIB_ControllerPIpAW_F16/copyright2 ==

== system ammclib_bam_S32K11x/GFLIB/F16/GFLIB_ControllerPIp_F16/copyright ==

== system ammclib_bam_S32K11x/GFLIB/F16/GFLIB_ControllerPIp_F16/copyright2 ==

== system ammclib_bam_S32K11x/GFLIB/F16/GFLIB_ControllerPIrAW_F16/copyright ==

== system ammclib_bam_S32K11x/GFLIB/F16/GFLIB_ControllerPIrAW_F16/copyright2 ==

== system ammclib_bam_S32K11x/GFLIB/F16/GFLIB_ControllerPIr_F16/copyright ==

== system ammclib_bam_S32K11x/GFLIB/F16/GFLIB_ControllerPIr_F16/copyright2 ==

== system ammclib_bam_S32K11x/GFLIB/F16/GFLIB_Cos_F16/copyright ==

== system ammclib_bam_S32K11x/GFLIB/F16/GFLIB_Cos_F16/copyright2 ==

== system ammclib_bam_S32K11x/GFLIB/F16/GFLIB_Hyst_F16/copyright ==

== system ammclib_bam_S32K11x/GFLIB/F16/GFLIB_Hyst_F16/copyright2 ==

== system ammclib_bam_S32K11x/GFLIB/F16/GFLIB_IntegratorTR_F16/copyright ==

== system ammclib_bam_S32K11x/GFLIB/F16/GFLIB_IntegratorTR_F16/copyright2 ==

== system ammclib_bam_S32K11x/GFLIB/F16/GFLIB_Limit_F16/copyright ==

== system ammclib_bam_S32K11x/GFLIB/F16/GFLIB_Limit_F16/copyright2 ==

== system ammclib_bam_S32K11x/GFLIB/F16/GFLIB_LowerLimit_F16/copyright ==

== system ammclib_bam_S32K11x/GFLIB/F16/GFLIB_LowerLimit_F16/copyright2 ==

== system ammclib_bam_S32K11x/GFLIB/F16/GFLIB_Lut1D_F16/copyright ==

== system ammclib_bam_S32K11x/GFLIB/F16/GFLIB_Lut1D_F16/copyright2 ==

== system ammclib_bam_S32K11x/GFLIB/F16/GFLIB_Lut2D_F16/copyright ==

== system ammclib_bam_S32K11x/GFLIB/F16/GFLIB_Lut2D_F16/copyright2 ==

== system ammclib_bam_S32K11x/GFLIB/F16/GFLIB_Ramp_F16/copyright ==

== system ammclib_bam_S32K11x/GFLIB/F16/GFLIB_Ramp_F16/copyright2 ==

== system ammclib_bam_S32K11x/GFLIB/F16/GFLIB_Sign_F16/copyright ==

== system ammclib_bam_S32K11x/GFLIB/F16/GFLIB_Sign_F16/copyright2 ==

== system ammclib_bam_S32K11x/GFLIB/F16/GFLIB_SinCos_F16/copyright ==

== system ammclib_bam_S32K11x/GFLIB/F16/GFLIB_SinCos_F16/copyright2 ==

== system ammclib_bam_S32K11x/GFLIB/F16/GFLIB_Sin_F16/copyright ==

== system ammclib_bam_S32K11x/GFLIB/F16/GFLIB_Sin_F16/copyright2 ==

== system ammclib_bam_S32K11x/GFLIB/F16/GFLIB_Sqrt_F16/copyright ==

== system ammclib_bam_S32K11x/GFLIB/F16/GFLIB_Sqrt_F16/copyright2 ==

== system ammclib_bam_S32K11x/GFLIB/F16/GFLIB_Tan_F16/copyright ==

== system ammclib_bam_S32K11x/GFLIB/F16/GFLIB_Tan_F16/copyright2 ==

== system ammclib_bam_S32K11x/GFLIB/F16/GFLIB_UpperLimit_F16/copyright ==

== system ammclib_bam_S32K11x/GFLIB/F16/GFLIB_UpperLimit_F16/copyright2 ==

== system ammclib_bam_S32K11x/GFLIB/F16/GFLIB_VMin_F16/copyright ==

== system ammclib_bam_S32K11x/GFLIB/F16/GFLIB_VMin_F16/copyright2 ==

== system ammclib_bam_S32K11x/GFLIB/F16/GFLIB_VectorLimit_F16/copyright ==

== system ammclib_bam_S32K11x/GFLIB/F16/GFLIB_VectorLimit_F16/copyright2 ==

== system ammclib_bam_S32K11x/GFLIB/F32/GFLIB_Acos_F32/copyright ==

== system ammclib_bam_S32K11x/GFLIB/F32/GFLIB_Acos_F32/copyright2 ==

== system ammclib_bam_S32K11x/GFLIB/F32/GFLIB_Asin_F32/copyright ==

== system ammclib_bam_S32K11x/GFLIB/F32/GFLIB_Asin_F32/copyright2 ==

== system ammclib_bam_S32K11x/GFLIB/F32/GFLIB_AtanYXShifted_F32/copyright ==

== system ammclib_bam_S32K11x/GFLIB/F32/GFLIB_AtanYXShifted_F32/copyright2 ==

== system ammclib_bam_S32K11x/GFLIB/F32/GFLIB_AtanYX_F32/copyright ==

== system ammclib_bam_S32K11x/GFLIB/F32/GFLIB_AtanYX_F32/copyright2 ==

== system ammclib_bam_S32K11x/GFLIB/F32/GFLIB_Atan_F32/copyright ==

== system ammclib_bam_S32K11x/GFLIB/F32/GFLIB_Atan_F32/copyright2 ==

== system ammclib_bam_S32K11x/GFLIB/F32/GFLIB_ControllerPIDpAW_F32/copyright ==

== system ammclib_bam_S32K11x/GFLIB/F32/GFLIB_ControllerPIDpAW_F32/copyright2 ==

== system ammclib_bam_S32K11x/GFLIB/F32/GFLIB_ControllerPIpAW_F32/copyright ==

== system ammclib_bam_S32K11x/GFLIB/F32/GFLIB_ControllerPIpAW_F32/copyright2 ==

== system ammclib_bam_S32K11x/GFLIB/F32/GFLIB_ControllerPIp_F32/copyright ==

== system ammclib_bam_S32K11x/GFLIB/F32/GFLIB_ControllerPIp_F32/copyright2 ==

== system ammclib_bam_S32K11x/GFLIB/F32/GFLIB_ControllerPIrAW_F32/copyright ==

== system ammclib_bam_S32K11x/GFLIB/F32/GFLIB_ControllerPIrAW_F32/copyright2 ==

== system ammclib_bam_S32K11x/GFLIB/F32/GFLIB_ControllerPIr_F32/copyright ==

== system ammclib_bam_S32K11x/GFLIB/F32/GFLIB_ControllerPIr_F32/copyright2 ==

== system ammclib_bam_S32K11x/GFLIB/F32/GFLIB_Cos_F32/copyright ==

== system ammclib_bam_S32K11x/GFLIB/F32/GFLIB_Cos_F32/copyright2 ==

== system ammclib_bam_S32K11x/GFLIB/F32/GFLIB_Hyst_F32/copyright ==

== system ammclib_bam_S32K11x/GFLIB/F32/GFLIB_Hyst_F32/copyright2 ==

== system ammclib_bam_S32K11x/GFLIB/F32/GFLIB_IntegratorTR_F32/copyright ==

== system ammclib_bam_S32K11x/GFLIB/F32/GFLIB_IntegratorTR_F32/copyright2 ==

== system ammclib_bam_S32K11x/GFLIB/F32/GFLIB_Limit_F32/copyright ==

== system ammclib_bam_S32K11x/GFLIB/F32/GFLIB_Limit_F32/copyright2 ==

== system ammclib_bam_S32K11x/GFLIB/F32/GFLIB_LowerLimit_F32/copyright ==

== system ammclib_bam_S32K11x/GFLIB/F32/GFLIB_LowerLimit_F32/copyright2 ==

== system ammclib_bam_S32K11x/GFLIB/F32/GFLIB_Lut1D_F32/copyright ==

== system ammclib_bam_S32K11x/GFLIB/F32/GFLIB_Lut1D_F32/copyright2 ==

== system ammclib_bam_S32K11x/GFLIB/F32/GFLIB_Lut2D_F32/copyright ==

== system ammclib_bam_S32K11x/GFLIB/F32/GFLIB_Lut2D_F32/copyright2 ==

== system ammclib_bam_S32K11x/GFLIB/F32/GFLIB_Ramp_F32/copyright ==

== system ammclib_bam_S32K11x/GFLIB/F32/GFLIB_Ramp_F32/copyright2 ==

== system ammclib_bam_S32K11x/GFLIB/F32/GFLIB_Sign_F32/copyright ==

== system ammclib_bam_S32K11x/GFLIB/F32/GFLIB_Sign_F32/copyright2 ==

== system ammclib_bam_S32K11x/GFLIB/F32/GFLIB_SinCos_F32/copyright ==

== system ammclib_bam_S32K11x/GFLIB/F32/GFLIB_SinCos_F32/copyright2 ==

== system ammclib_bam_S32K11x/GFLIB/F32/GFLIB_Sin_F32/copyright ==

== system ammclib_bam_S32K11x/GFLIB/F32/GFLIB_Sin_F32/copyright2 ==

== system ammclib_bam_S32K11x/GFLIB/F32/GFLIB_Sqrt_F32/copyright ==

== system ammclib_bam_S32K11x/GFLIB/F32/GFLIB_Sqrt_F32/copyright2 ==

== system ammclib_bam_S32K11x/GFLIB/F32/GFLIB_Tan_F32/copyright ==

== system ammclib_bam_S32K11x/GFLIB/F32/GFLIB_Tan_F32/copyright2 ==

== system ammclib_bam_S32K11x/GFLIB/F32/GFLIB_UpperLimit_F32/copyright ==

== system ammclib_bam_S32K11x/GFLIB/F32/GFLIB_UpperLimit_F32/copyright2 ==

== system ammclib_bam_S32K11x/GFLIB/F32/GFLIB_VMin_F32/copyright ==

== system ammclib_bam_S32K11x/GFLIB/F32/GFLIB_VMin_F32/copyright2 ==

== system ammclib_bam_S32K11x/GFLIB/F32/GFLIB_VectorLimit_F32/copyright ==

== system ammclib_bam_S32K11x/GFLIB/F32/GFLIB_VectorLimit_F32/copyright2 ==

== system ammclib_bam_S32K11x/GMCLIB/F16/GMCLIB_BetaProjection3Ph_F16/copyright ==

== system ammclib_bam_S32K11x/GMCLIB/F16/GMCLIB_BetaProjection3Ph_F16/copyright2 ==

== system ammclib_bam_S32K11x/GMCLIB/F16/GMCLIB_BetaProjection_F16/copyright ==

== system ammclib_bam_S32K11x/GMCLIB/F16/GMCLIB_BetaProjection_F16/copyright2 ==

== system ammclib_bam_S32K11x/GMCLIB/F16/GMCLIB_ClarkInv_F16/copyright ==

== system ammclib_bam_S32K11x/GMCLIB/F16/GMCLIB_ClarkInv_F16/copyright2 ==

== system ammclib_bam_S32K11x/GMCLIB/F16/GMCLIB_Clark_F16/copyright ==

== system ammclib_bam_S32K11x/GMCLIB/F16/GMCLIB_Clark_F16/copyright2 ==

== system ammclib_bam_S32K11x/GMCLIB/F16/GMCLIB_DecouplingPMSM_F16/copyright ==

== system ammclib_bam_S32K11x/GMCLIB/F16/GMCLIB_DecouplingPMSM_F16/copyright2 ==

== system ammclib_bam_S32K11x/GMCLIB/F16/GMCLIB_ElimDcBusRip_F16/copyright ==

== system ammclib_bam_S32K11x/GMCLIB/F16/GMCLIB_ElimDcBusRip_F16/copyright2 ==

== system ammclib_bam_S32K11x/GMCLIB/F16/GMCLIB_ParkInv_F16/copyright ==

== system ammclib_bam_S32K11x/GMCLIB/F16/GMCLIB_ParkInv_F16/copyright2 ==

== system ammclib_bam_S32K11x/GMCLIB/F16/GMCLIB_Park_F16/copyright ==

== system ammclib_bam_S32K11x/GMCLIB/F16/GMCLIB_Park_F16/copyright2 ==

== system ammclib_bam_S32K11x/GMCLIB/F16/GMCLIB_PwmIct_F16/copyright ==

== system ammclib_bam_S32K11x/GMCLIB/F16/GMCLIB_PwmIct_F16/copyright2 ==

== system ammclib_bam_S32K11x/GMCLIB/F16/GMCLIB_SvmSci_F16/copyright ==

== system ammclib_bam_S32K11x/GMCLIB/F16/GMCLIB_SvmSci_F16/copyright2 ==

== system ammclib_bam_S32K11x/GMCLIB/F16/GMCLIB_SvmStd_F16/copyright ==

== system ammclib_bam_S32K11x/GMCLIB/F16/GMCLIB_SvmStd_F16/copyright2 ==

== system ammclib_bam_S32K11x/GMCLIB/F16/GMCLIB_SvmU0n_F16/copyright ==

== system ammclib_bam_S32K11x/GMCLIB/F16/GMCLIB_SvmU0n_F16/copyright2 ==

== system ammclib_bam_S32K11x/GMCLIB/F16/GMCLIB_SvmU7n_F16/copyright ==

== system ammclib_bam_S32K11x/GMCLIB/F16/GMCLIB_SvmU7n_F16/copyright2 ==

== system ammclib_bam_S32K11x/GMCLIB/F16/GMCLIB_VRot_F16/copyright ==

== system ammclib_bam_S32K11x/GMCLIB/F16/GMCLIB_VRot_F16/copyright2 ==

== system ammclib_bam_S32K11x/GMCLIB/F16/GMCLIB_VUnit_F16/copyright ==

== system ammclib_bam_S32K11x/GMCLIB/F16/GMCLIB_VUnit_F16/copyright2 ==

== system ammclib_bam_S32K11x/GMCLIB/F16/GMCLIB_Vpol2xy_F16/copyright ==

== system ammclib_bam_S32K11x/GMCLIB/F16/GMCLIB_Vpol2xy_F16/copyright2 ==

== system ammclib_bam_S32K11x/GMCLIB/F16/GMCLIB_Vxy2pol_F16/copyright ==

== system ammclib_bam_S32K11x/GMCLIB/F16/GMCLIB_Vxy2pol_F16/copyright2 ==

== system ammclib_bam_S32K11x/GMCLIB/F32/GMCLIB_BetaProjection3Ph_F32/copyright ==

== system ammclib_bam_S32K11x/GMCLIB/F32/GMCLIB_BetaProjection3Ph_F32/copyright2 ==

== system ammclib_bam_S32K11x/GMCLIB/F32/GMCLIB_BetaProjection_F32/copyright ==

== system ammclib_bam_S32K11x/GMCLIB/F32/GMCLIB_BetaProjection_F32/copyright2 ==

== system ammclib_bam_S32K11x/GMCLIB/F32/GMCLIB_ClarkInv_F32/copyright ==

== system ammclib_bam_S32K11x/GMCLIB/F32/GMCLIB_ClarkInv_F32/copyright2 ==

== system ammclib_bam_S32K11x/GMCLIB/F32/GMCLIB_Clark_F32/copyright ==

== system ammclib_bam_S32K11x/GMCLIB/F32/GMCLIB_Clark_F32/copyright2 ==

== system ammclib_bam_S32K11x/GMCLIB/F32/GMCLIB_DecouplingPMSM_F32/copyright ==

== system ammclib_bam_S32K11x/GMCLIB/F32/GMCLIB_DecouplingPMSM_F32/copyright2 ==

== system ammclib_bam_S32K11x/GMCLIB/F32/GMCLIB_ElimDcBusRip_F32/copyright ==

== system ammclib_bam_S32K11x/GMCLIB/F32/GMCLIB_ElimDcBusRip_F32/copyright2 ==

== system ammclib_bam_S32K11x/GMCLIB/F32/GMCLIB_ParkInv_F32/copyright ==

== system ammclib_bam_S32K11x/GMCLIB/F32/GMCLIB_ParkInv_F32/copyright2 ==

== system ammclib_bam_S32K11x/GMCLIB/F32/GMCLIB_Park_F32/copyright ==

== system ammclib_bam_S32K11x/GMCLIB/F32/GMCLIB_Park_F32/copyright2 ==

== system ammclib_bam_S32K11x/GMCLIB/F32/GMCLIB_PwmIct_F32/copyright ==

== system ammclib_bam_S32K11x/GMCLIB/F32/GMCLIB_PwmIct_F32/copyright2 ==

== system ammclib_bam_S32K11x/GMCLIB/F32/GMCLIB_SvmSci_F32/copyright ==

== system ammclib_bam_S32K11x/GMCLIB/F32/GMCLIB_SvmSci_F32/copyright2 ==

== system ammclib_bam_S32K11x/GMCLIB/F32/GMCLIB_SvmStd_F32/copyright ==

== system ammclib_bam_S32K11x/GMCLIB/F32/GMCLIB_SvmStd_F32/copyright2 ==

== system ammclib_bam_S32K11x/GMCLIB/F32/GMCLIB_SvmU0n_F32/copyright ==

== system ammclib_bam_S32K11x/GMCLIB/F32/GMCLIB_SvmU0n_F32/copyright2 ==

== system ammclib_bam_S32K11x/GMCLIB/F32/GMCLIB_SvmU7n_F32/copyright ==

== system ammclib_bam_S32K11x/GMCLIB/F32/GMCLIB_SvmU7n_F32/copyright2 ==

== system ammclib_bam_S32K11x/GMCLIB/F32/GMCLIB_VRot_F32/copyright ==

== system ammclib_bam_S32K11x/GMCLIB/F32/GMCLIB_VRot_F32/copyright2 ==

== system ammclib_bam_S32K11x/GMCLIB/F32/GMCLIB_VUnit_F32/copyright ==

== system ammclib_bam_S32K11x/GMCLIB/F32/GMCLIB_VUnit_F32/copyright2 ==

== system ammclib_bam_S32K11x/GMCLIB/F32/GMCLIB_Vpol2xy_F32/copyright ==

== system ammclib_bam_S32K11x/GMCLIB/F32/GMCLIB_Vpol2xy_F32/copyright2 ==

== system ammclib_bam_S32K11x/GMCLIB/F32/GMCLIB_Vxy2pol_F32/copyright ==

== system ammclib_bam_S32K11x/GMCLIB/F32/GMCLIB_Vxy2pol_F32/copyright2 ==

== system ammclib_bam_S32K11x/MLIB/F16/MLIB_AbsSat_F16/copyright ==

== system ammclib_bam_S32K11x/MLIB/F16/MLIB_AbsSat_F16/copyright2 ==

== system ammclib_bam_S32K11x/MLIB/F16/MLIB_Abs_F16/copyright ==

== system ammclib_bam_S32K11x/MLIB/F16/MLIB_Abs_F16/copyright2 ==

== system ammclib_bam_S32K11x/MLIB/F16/MLIB_AddSat_F16/copyright ==

== system ammclib_bam_S32K11x/MLIB/F16/MLIB_AddSat_F16/copyright2 ==

== system ammclib_bam_S32K11x/MLIB/F16/MLIB_Add_F16/copyright ==

== system ammclib_bam_S32K11x/MLIB/F16/MLIB_Add_F16/copyright2 ==

== system ammclib_bam_S32K11x/MLIB/F16/MLIB_ConvertPU_F16F32/copyright ==

== system ammclib_bam_S32K11x/MLIB/F16/MLIB_ConvertPU_F16F32/copyright2 ==

== system ammclib_bam_S32K11x/MLIB/F16/MLIB_Convert_F16F32/copyright ==

== system ammclib_bam_S32K11x/MLIB/F16/MLIB_Convert_F16F32/copyright2 ==

== system ammclib_bam_S32K11x/MLIB/F16/MLIB_DivSat_F16/copyright ==

== system ammclib_bam_S32K11x/MLIB/F16/MLIB_DivSat_F16/copyright2 ==

== system ammclib_bam_S32K11x/MLIB/F16/MLIB_Div_F16/copyright ==

== system ammclib_bam_S32K11x/MLIB/F16/MLIB_Div_F16/copyright2 ==

== system ammclib_bam_S32K11x/MLIB/F16/MLIB_MacSat_F16/copyright ==

== system ammclib_bam_S32K11x/MLIB/F16/MLIB_MacSat_F16/copyright2 ==

== system ammclib_bam_S32K11x/MLIB/F16/MLIB_Mac_F16/copyright ==

== system ammclib_bam_S32K11x/MLIB/F16/MLIB_Mac_F16/copyright2 ==

== system ammclib_bam_S32K11x/MLIB/F16/MLIB_Mnac_F16/copyright ==

== system ammclib_bam_S32K11x/MLIB/F16/MLIB_Mnac_F16/copyright2 ==

== system ammclib_bam_S32K11x/MLIB/F16/MLIB_Msu_F16/copyright ==

== system ammclib_bam_S32K11x/MLIB/F16/MLIB_Msu_F16/copyright2 ==

== system ammclib_bam_S32K11x/MLIB/F16/MLIB_MulSat_F16/copyright ==

== system ammclib_bam_S32K11x/MLIB/F16/MLIB_MulSat_F16/copyright2 ==

== system ammclib_bam_S32K11x/MLIB/F16/MLIB_Mul_F16/copyright ==

== system ammclib_bam_S32K11x/MLIB/F16/MLIB_Mul_F16/copyright2 ==

== system ammclib_bam_S32K11x/MLIB/F16/MLIB_NegSat_F16/copyright ==

== system ammclib_bam_S32K11x/MLIB/F16/MLIB_NegSat_F16/copyright2 ==

== system ammclib_bam_S32K11x/MLIB/F16/MLIB_Neg_F16/copyright ==

== system ammclib_bam_S32K11x/MLIB/F16/MLIB_Neg_F16/copyright2 ==

== system ammclib_bam_S32K11x/MLIB/F16/MLIB_Norm_F16/copyright ==

== system ammclib_bam_S32K11x/MLIB/F16/MLIB_Norm_F16/copyright2 ==

== system ammclib_bam_S32K11x/MLIB/F16/MLIB_RndSat_F16F32/copyright ==

== system ammclib_bam_S32K11x/MLIB/F16/MLIB_RndSat_F16F32/copyright2 ==

== system ammclib_bam_S32K11x/MLIB/F16/MLIB_Round_F16/copyright ==

== system ammclib_bam_S32K11x/MLIB/F16/MLIB_Round_F16/copyright2 ==

== system ammclib_bam_S32K11x/MLIB/F16/MLIB_ShBiSat_F16/copyright ==

== system ammclib_bam_S32K11x/MLIB/F16/MLIB_ShBiSat_F16/copyright2 ==

== system ammclib_bam_S32K11x/MLIB/F16/MLIB_ShBi_F16/copyright ==

== system ammclib_bam_S32K11x/MLIB/F16/MLIB_ShBi_F16/copyright2 ==

== system ammclib_bam_S32K11x/MLIB/F16/MLIB_ShLSat_F16/copyright ==

== system ammclib_bam_S32K11x/MLIB/F16/MLIB_ShLSat_F16/copyright2 ==

== system ammclib_bam_S32K11x/MLIB/F16/MLIB_ShL_F16/copyright ==

== system ammclib_bam_S32K11x/MLIB/F16/MLIB_ShL_F16/copyright2 ==

== system ammclib_bam_S32K11x/MLIB/F16/MLIB_ShR_F16/copyright ==

== system ammclib_bam_S32K11x/MLIB/F16/MLIB_ShR_F16/copyright2 ==

== system ammclib_bam_S32K11x/MLIB/F16/MLIB_SubSat_F16/copyright ==

== system ammclib_bam_S32K11x/MLIB/F16/MLIB_SubSat_F16/copyright2 ==

== system ammclib_bam_S32K11x/MLIB/F16/MLIB_Sub_F16/copyright ==

== system ammclib_bam_S32K11x/MLIB/F16/MLIB_Sub_F16/copyright2 ==

== system ammclib_bam_S32K11x/MLIB/F16/MLIB_VAdd_F16/copyright ==

== system ammclib_bam_S32K11x/MLIB/F16/MLIB_VAdd_F16/copyright2 ==

== system ammclib_bam_S32K11x/MLIB/F16/MLIB_VMac_F16/copyright ==

== system ammclib_bam_S32K11x/MLIB/F16/MLIB_VMac_F16/copyright2 ==

== system ammclib_bam_S32K11x/MLIB/F16/MLIB_VScale_F16/copyright ==

== system ammclib_bam_S32K11x/MLIB/F16/MLIB_VScale_F16/copyright2 ==

== system ammclib_bam_S32K11x/MLIB/F16/MLIB_VSub_F16/copyright ==

== system ammclib_bam_S32K11x/MLIB/F16/MLIB_VSub_F16/copyright2 ==

== system ammclib_bam_S32K11x/MLIB/F32/MLIB_AbsSat_F32/copyright ==

== system ammclib_bam_S32K11x/MLIB/F32/MLIB_AbsSat_F32/copyright2 ==

== system ammclib_bam_S32K11x/MLIB/F32/MLIB_Abs_F32/copyright ==

== system ammclib_bam_S32K11x/MLIB/F32/MLIB_Abs_F32/copyright2 ==

== system ammclib_bam_S32K11x/MLIB/F32/MLIB_AddSat_F32/copyright ==

== system ammclib_bam_S32K11x/MLIB/F32/MLIB_AddSat_F32/copyright2 ==

== system ammclib_bam_S32K11x/MLIB/F32/MLIB_Add_F32/copyright ==

== system ammclib_bam_S32K11x/MLIB/F32/MLIB_Add_F32/copyright2 ==

== system ammclib_bam_S32K11x/MLIB/F32/MLIB_ConvertPU_F32F16/copyright ==

== system ammclib_bam_S32K11x/MLIB/F32/MLIB_ConvertPU_F32F16/copyright2 ==

== system ammclib_bam_S32K11x/MLIB/F32/MLIB_Convert_F32F16/copyright ==

== system ammclib_bam_S32K11x/MLIB/F32/MLIB_Convert_F32F16/copyright2 ==

== system ammclib_bam_S32K11x/MLIB/F32/MLIB_DivSat_F32/copyright ==

== system ammclib_bam_S32K11x/MLIB/F32/MLIB_DivSat_F32/copyright2 ==

== system ammclib_bam_S32K11x/MLIB/F32/MLIB_Div_F32/copyright ==

== system ammclib_bam_S32K11x/MLIB/F32/MLIB_Div_F32/copyright2 ==
